simulink model "canyongenerator"  (Simulink 9.1)
settings: Solver=ode45  StartTime=0.0  StopTime=100  RelTol=1e-3  EnableMultiTasking=on
values from neighbouring files (symbols this model uses):
  K = -K    [FindF16DynamicsCanyon.m]
  sys_rr = ss(A_rr,B_rr,C_rr,D_rr)    [FindF16DynamicsCanyon.m]
  trim_control_lo = [-2.46068617229 3.21143579128e-16 2.79661206579e-15]    [chap5data.mat]    (also in data.mat)
  trim_thrust_lo = 2120.62144782    [chap5data.mat]    (also in data.mat)
  velocity = input('Enter the velocity for the simulation (ft/s):  ')    [FindF16Dynamics.m]    (also in FindF16DynamicsCanyon.m = 300; chap5data.mat = 500; data.mat = 500; trim_F16.m = vel)
libraries: aerolibconvert2 x5
settings Model: Creator=tlombaerts  LastModifiedBy=benja
settings DataIOCC: SignalLoggingSaveFormat=ModelDataLogs
settings OptimizationCC: ExpressionDepthLimit=2147483647  InitFltsAndDblsToZero=on
settings DebuggingCC: SaveWithParameterizedLinksMsg=none  SignalResolutionControl=TryResolveAllWithWarning  SolverPrmCheckMsg=warning  FcnCallInpInsideContextMsg=warning  StateNameClashWarn=warning
settings GRTTargetCC: TargetFcnLib=ansi_tfl_tmw.mat

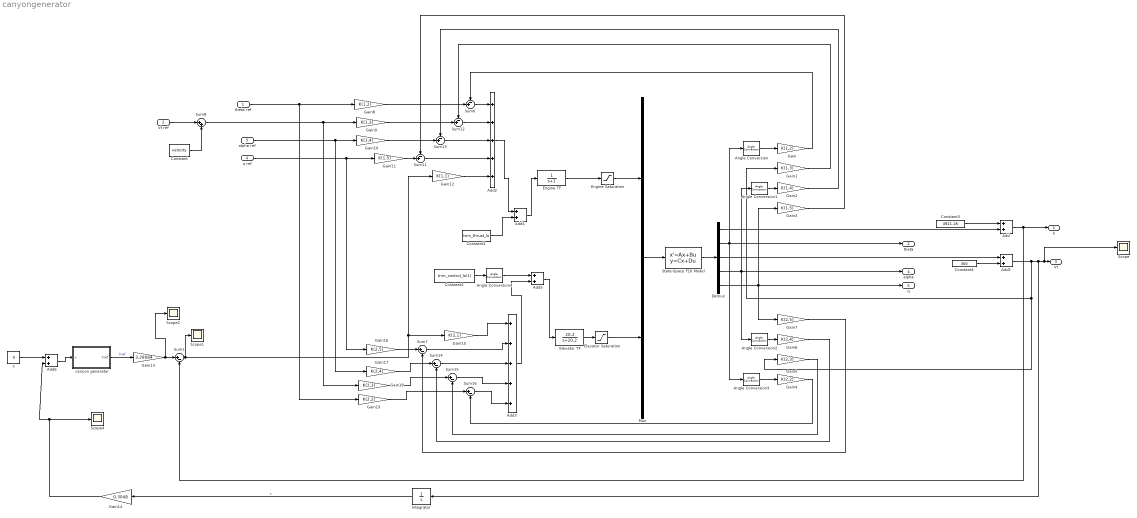
== system canyongenerator ==
  "theta ref " : Inport
  Vt ref : Inport  Port=2
  alpha ref : Inport  Port=3
  q ref : Inport  Port=4
  Add{,1,4..6} (5 alike) : Sum
  Add2 : Sum  Inputs=+++++
  Add3 : Sum  Inputs=+++++
  Angle Conversion{,1..4} (5 alike) : aerolibconvert2/Angle Conversion  IU=deg  OU=rad
  Constant : Constant  Value=velocity
  Constant1 : Constant  Value=trim_thrust_lo
  Constant2 : Constant  Value=trim_control_lo(1)
  Constant3 : Constant  Value=4921.26
  Constant4 : Constant  Value=300  VectorParams1D=off  SampleTime=-1
  Demux : Demux  Outputs=5
  Elevator Saturation : Saturate  UpperLimit=0.436332  LowerLimit=-0.436332
  Elevator TF : TransferFcn  Numerator=[20.2]  Denominator=[1 20.2]
  Engine Saturation : Saturate  UpperLimit=19000  LowerLimit=1000
  Engine TF : TransferFcn  Denominator=[1 1]
  Gain : Gain  Gain=K(1,2)
  Gain1 : Gain  Gain=K(1,3)
  Gain10 : Gain  Gain=K(1,4)
  Gain11 : Gain  Gain=K(1,5)
  Gain12 : Gain  Gain=K(1,1)
  Gain13 : Gain  Gain=3.28084
  Gain14 : Gain  Gain=0.3048
  Gain15 : Gain  Gain=K(2,1)
  Gain16 : Gain  Gain=K(2,5)
  Gain17 : Gain  Gain=K(2,4)
  Gain18 : Gain  Gain=K(2,3)
  Gain19 : Gain  Gain=K(2,2)
  Gain2 : Gain  Gain=K(1,4)
  Gain3 : Gain  Gain=K(1,5)
  Gain4 : Gain  Gain=K(2,2)
  Gain5 : Gain  Gain=K(2,3)
  Gain6 : Gain  Gain=K(2,4)
  Gain7 : Gain  Gain=K(2,5)
  Gain8 : Gain  Gain=K(1,2)
  Gain9 : Gain  Gain=K(1,3)
  Integrator : Integrator
  Mux : Mux  Inputs=2
  Scope{,1..2,4} (4 alike) : Scope
  State-Space F16 Model : StateSpace  A=sys_rr.A  B=sys_rr.B  C=sys_rr.C  D=sys_rr.D  InitialCondition=0
  Sum{1,7,14..16} (5 alike) : Sum  Inputs=|+-
  Sum{6,11..13} (4 alike) : Sum  Inputs=-+|
  Sum8 : Sum  Inputs=|++
  canyon generator : Subsystem
      mask Display: image(imread('refalt.jpg'))
  x : Constant  Value=0
  h : Outport
  theta : Outport  Port=2
  Vt : Outport  Port=3
  " alpha" : Outport  Port=4
  q : Outport  Port=5
  wires:
  Mux/1 -> State-Space F16 Model/1
  State-Space F16 Model/1 -> Demux/1
  Demux/2 -> Angle Conversion3/1, Angle Conversion/1, theta/1
  Demux/3 -> Add1/1
  Demux/4 -> Angle Conversion2/1, " alpha"/1, Angle Conversion1/1
  Demux/5 -> Gain7/1, q/1, Gain3/1
  Elevator Saturation/1 -> Mux/2
  Engine Saturation/1 -> Mux/1
  Engine TF/1 -> Engine Saturation/1
  Elevator TF/1 -> Elevator Saturation/1
  Integrator/1 -> Gain14/1  "x"
  Gain/1 -> Sum6/1
  Gain2/1 -> Sum13/1
  Gain3/1 -> Sum11/1
  Gain7/1 -> Sum7/2
  Gain5/1 -> Sum15/2
  Gain6/1 -> Sum14/2
  Add2/1 -> Add4/1
  Add3/1 -> Add5/2
  Sum6/1 -> Add2/1
  Sum7/1 -> Add3/2
  Vt ref/1 -> Sum8/1
  Gain13/1 -> Scope2/1, Sum1/1
  Gain14/1 -> Add6/2, Scope4/1
  Gain12/1 -> Add2/5
  Gain15/1 -> Add3/1
  Sum1/1 -> Scope1/1, Gain15/1, Gain12/1
  x/1 -> Add6/1
  Angle Conversion/1 -> Gain/1
  Angle Conversion1/1 -> Gain2/1
  Angle Conversion3/1 -> Gain4/1
  Angle Conversion2/1 -> Gain6/1
  Constant/1 -> Sum8/2
  canyon generator/1(href) -> Gain13/1  "href"
  Demux/1 -> Add/2
  "theta ref "/1 -> Gain8/1, Gain19/1
  Sum13/1 -> Add2/3
  Sum11/1 -> Add2/4
  Sum12/1 -> Add2/2
  Gain1/1 -> Sum12/1
  Sum8/1 -> Gain9/1, Gain18/1
  alpha ref/1 -> Gain10/1, Gain17/1
  q ref/1 -> Gain11/1, Gain16/1
  Sum16/1 -> Add3/5
  Sum15/1 -> Add3/4
  Sum14/1 -> Add3/3
  Gain4/1 -> Sum16/2
  Add/1 -> h/1, Sum1/2
  Constant3/1 -> Add/1
  Add1/1 -> Gain1/1, Gain5/1, Integrator/1, Scope/1, Vt/1
  Constant4/1 -> Add1/2
  Add4/1 -> Engine TF/1
  Add5/1 -> Elevator TF/1
  Constant1/1 -> Add4/2
  Constant2/1 -> Angle Conversion4/1
  Angle Conversion4/1 -> Add5/1
  Gain8/1 -> Sum6/2
  Gain9/1 -> Sum12/2
  Gain10/1 -> Sum13/2
  Gain11/1 -> Sum11/2
  Gain16/1 -> Sum7/1
  Gain17/1 -> Sum14/1
  Gain18/1 -> Sum15/1
  Gain19/1 -> Sum16/1
  Add6/1 -> canyon generator/1(x)

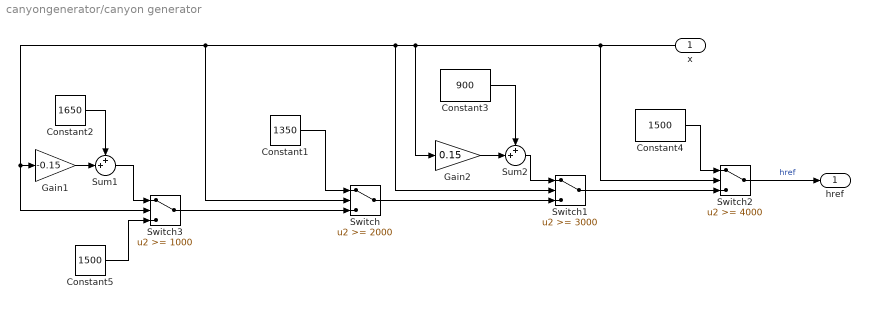
== system canyongenerator/canyon generator ==
  x : Inport
  Constant1 : Constant  Value=1350
  Constant2 : Constant  Value=1650
  Constant3 : Constant  Value=900
  Constant4 : Constant  Value=1500
  Constant5 : Constant  Value=1500
  Gain1 : Gain  Gain=-0.15
  Gain2 : Gain  Gain=0.15
  Sum1 : Sum  Inputs=++|
  Sum2 : Sum  Inputs=++|
  Switch : Switch  Threshold=2000  ZeroCross=off
  Switch1 : Switch  Threshold=3000  ZeroCross=off
  Switch2 : Switch  Threshold=4000  ZeroCross=off
  Switch3 : Switch  Threshold=1000  ZeroCross=off
  href : Outport
  wires:
  Constant1/1 -> Switch/1
  x/1 -> Switch2/2, Gain2/1, Switch1/2, Switch/2, Gain1/1, Switch3/2
  Switch/1 -> Switch1/3
  Gain2/1 -> Sum2/2
  Constant3/1 -> Sum2/1
  Sum2/1 -> Switch1/1
  Switch1/1 -> Switch2/3
  Constant4/1 -> Switch2/1
  Switch2/1 -> href/1  "href"
  Switch3/1 -> Switch/3
  Gain1/1 -> Sum1/2
  Constant2/1 -> Sum1/1
  Constant5/1 -> Switch3/3
  Sum1/1 -> Switch3/1
